simulink model "ballbeam_animation"  (Simulink 8.3)
settings: Solver=ode45  StartTime=0.0  StopTime=10  RelTol=1e-3
undefined symbols (not defined in the file or in its folder): drawBallBeam
libraries: simulink x1
settings Model: Creator=beard  LastModifiedBy=jhl48
settings OptimizationCC: ExpressionDepthLimit=2147483647  InitFltsAndDblsToZero=on
settings DebuggingCC: FcnCallInpInsideContextMsg=UseLocalSettings

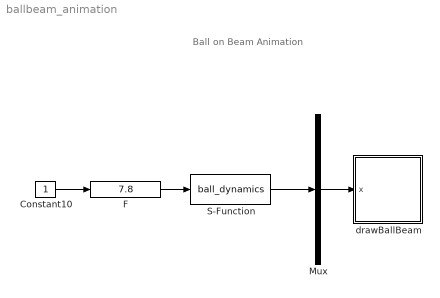
== system ballbeam_animation ==
  note: Ball on Beam Animation
  Constant10 : Constant
  F : simulink/Math Operations/Slider Gain  low=-100  gain=7.8  high=100
  Mux : Mux  Inputs=1
  S-Function : S-Function  FunctionName=ball_dynamics  Parameters=AP  EnableBusSupport=off
  drawBallBeam : Subsystem
      mask init:
      | % drawing parameters
      | L = 10;
      | R = 1;
      mask Display: image(imread('tv.jpg'))
  wires:
  Constant10/1 -> F/1
  Mux/1 -> drawBallBeam/1(x)
  F/1 -> S-Function/1
  S-Function/1 -> Mux/1

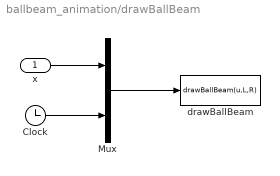
== system ballbeam_animation/drawBallBeam ==
  x : Inport
  Clock : Clock
  Mux : Mux  Inputs=2
  drawBallBeam : MATLABFcn  MATLABFcn=drawBallBeam(u,L,R)  OutputDimensions=0  SampleTime=0.001
  wires:
  Mux/1 -> drawBallBeam/1
  x/1 -> Mux/1
  Clock/1 -> Mux/2
